simulink model "Example1"  (R2014a)
settings: Solver=ode45  StartTime=0.0  StopTime=10.0  RelTol=1e-3
settings Model: Creator=matteo  LastModifiedBy=matteo
settings DebuggingCC: SolverPrmCheckMsg=none

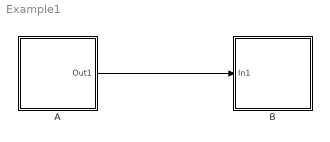
== system Example1 ==
  A : Subsystem
  B : Subsystem  Tag=monitoring
  wires:
  A/1(Out1) -> B/1(In1)

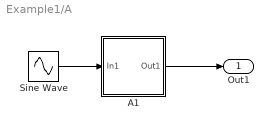
== system Example1/A ==
  A1 : Subsystem
  Sine Wave : Sin  SampleTime=0
  Out1 : Outport
  wires:
  Sine Wave/1 -> A1/1(In1)
  A1/1(Out1) -> Out1/1

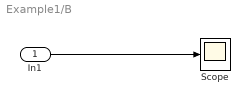
== system Example1/B ==
  In1 : Inport
  Scope : Scope
  wires:
  In1/1 -> Scope/1

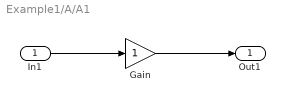
== system Example1/A/A1 ==
  In1 : Inport
  Gain : Gain
  Out1 : Outport
  wires:
  Gain/1 -> Out1/1
  In1/1 -> Gain/1
